simulink model "gatorKator_spectrum_visualization"  (Simulink 7.7)
settings: Solver=FixedStepDiscrete  StartTime=21e-3  StopTime=inf  RelTol=1e-3
undefined symbols (not defined in the file or in its folder): jet
libraries: dspsnks4 x5, dspspect3 x2, dspmtrx3 x2, dspmathops x2, commchan3 x1, dsparch4 x1, dspsrcs4 x1, dspstat3 x1, dspindex x1
settings Model: Creator=staticd  LastModifiedBy=staticd

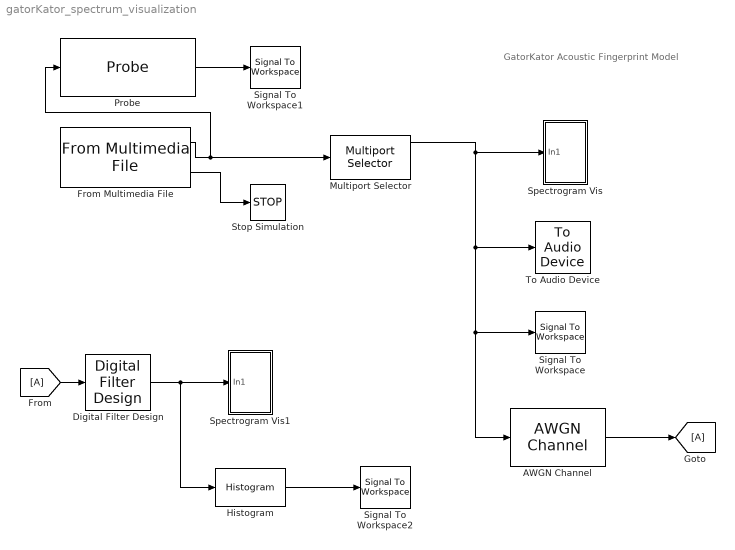
== system gatorKator_spectrum_visualization ==
  note: GatorKator Acoustic Fingerprint Model
  AWGN Channel : commchan3/AWGN Channel  SystemSampleTime=-1  InputProcessing=Columns as channels (frame based)  seed=67  noiseMode="Signal to noise ratio  (SNR)"  EbNodB=10  EsNodB=10  SNRdB=-20  bitsPerSym=1  Ps=1  Tsym=1  variance=1
  Digital Filter Design : dsparch4/Digital Filter Design  SystemSampleTime=-1  mwdsp_browser_bugfix_var=off
  From Multimedia File : dspsrcs4/From Multimedia File  inputFilename=C:\Users\staticd\Documents\My Dropbox\forLeo (2)\project\sample_data\deep_growl_converted.wav  loop=on  numPlays=inf  outputStreams=Audio only  videoDataType=single  audioDataType=double  inheritSampleTime=on  userDefinedSampleTime=1/30  noAudioOutput=off  isIntensityVideo=off  fourcc=RGB  colorVideoFormat=Separate color signals  outputEOF=on  dataOrg=Column-major  audioFrameSize=1024  computeAudioFrameSize=off
  Histogram : dspstat3/Histogram  umin=-1  umax=1  nbins=1e3  normalized=off  run=off  reset=on  trigtype=None  operateOver=Entire input  Dimension=1  colComp=on  roundingMode=Floor  overflowMode=off
  Multiport Selector : dspindex/Multiport Selector  rowsOrCols=Columns  idxCellArray={ 4, [1:2 5], [7; 8], 10:-1:6 }  idxErrMode=Clip Index
  Probe : Probe  ProbeWidth=off  ProbeComplexSignal=off
  Signal To Workspace : SignalToWorkspace  VariableName=yout  SaveFormat=Array  Save2DMode=2-D array (concatenate along first dimension)
      settings: CopyFcn=dspblkcopystw(gcbh);
  Signal To Workspace1 : SignalToWorkspace  VariableName=T  SaveFormat=Array  Save2DMode=2-D array (concatenate along first dimension)
      settings: CopyFcn=dspblkcopystw(gcbh);
  Signal To Workspace2 : SignalToWorkspace  VariableName=T1  SaveFormat=Array  Save2DMode=2-D array (concatenate along first dimension)
      settings: CopyFcn=dspblkcopystw(gcbh);
  Spectrogram Vis : Subsystem
  Spectrogram Vis1 : Subsystem
  Stop Simulation : Stop
  To Audio Device : dspsnks4/To Audio Device  deviceName=Default  inheritSampleRate=on  sampleRate=44100  deviceDatatype=Determine from input data type  autoBufferSize=on  bufferSize=4096  queueDuration=1.0
  wires:
  From Multimedia File/1 -> Probe/1, Multiport Selector/1
  Multiport Selector/1 -> Spectrogram Vis/1(In1), To Audio Device/1, Signal To Workspace/1, AWGN Channel/1
  From Multimedia File/2 -> Stop Simulation/1
  Probe/1 -> Signal To Workspace1/1
  [A] -> Digital Filter Design/1
  Digital Filter Design/1 -> Spectrogram Vis1/1(In1), Histogram/1
  Histogram/1 -> Signal To Workspace2/1
  AWGN Channel/1 -> [A]

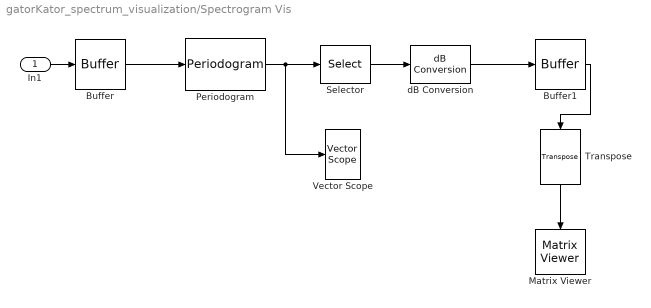
== system gatorKator_spectrum_visualization/Spectrogram Vis ==
  In1 : Inport
  Buffer : Buffer  N=256  TreatMby1Signals=One channel
  Buffer1 : Buffer  V=60  ic=-1
  Matrix Viewer : dspsnks4/Matrix Viewer  ImageParams=off  CMapStr=jet(256)  AxisColorbar=on  AxisParams=off  AxisOrigin=Lower left corner  XLabel=Time Index  YLabel=Frequency Index  ZLabel=dB Magnitude  FigPos=[50 530 1300 320]  AxisZoom=off
      settings: YMin=-80  YMax=10
  Periodogram : dspspect3/Periodogram  SystemSampleTime=-1  measurement=Power spectral density  wintype=Hamming  Rs=50  beta=5  winsamp=Periodic  inheritFFT=on  fftsize=256  navg=1  inheritTs=on  Ts=1
  Selector : Selector  InputPortWidth=256  IndexOptions=Index vector (dialog)  Indices=[1:128]  OutputSizes=1
  Transpose : dspmtrx3/Transpose  SystemSampleTime=-1  Hermitian=off  overflowFlag=off
  Vector Scope : dspsnks4/Vector Scope  ScopeProperties=on  Domain=Frequency  HorizSpan=1  DisplayProperties=off  AxisGrid=on  Memory=off  FrameNumber=on  AxisLegend=off  AxisZoom=off  OpenScopeAtSimStart=on  OpenScopeImmediately=off  FigPos=[50 110 1300 320]  AxisProperties=off  XUnits=Hertz  XRange=[0...Fs/2]  InheritXIncr=on  XIncr=1  XLabel=Time  XLimit=User-defined  XMin=0  XMax=3.5e3  XStart=0  YUnits=dB  YLabel=Magnitude, dB  LineProperties=off  XAxisParamsVer=6.9
      settings: YMin=-80  YMax=10
  dB Conversion : dspmathops/dB Conversion  SystemSampleTime=-1  dBtype=dB  intype=Power  R=1  fuzz=on
  wires:
  In1/1 -> Buffer/1
  Transpose/1 -> Matrix Viewer/1
  Buffer1/1 -> Transpose/1
  dB Conversion/1 -> Buffer1/1
  Selector/1 -> dB Conversion/1
  Periodogram/1 -> Vector Scope/1, Selector/1
  Buffer/1 -> Periodogram/1

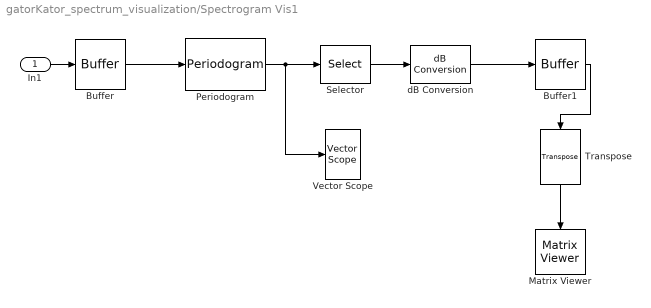
== system gatorKator_spectrum_visualization/Spectrogram Vis1 ==
  In1 : Inport
  Buffer : Buffer  N=256  TreatMby1Signals=One channel
  Buffer1 : Buffer  V=60  ic=-1
  Matrix Viewer : dspsnks4/Matrix Viewer  ImageParams=off  CMapStr=jet(256)  AxisColorbar=on  AxisParams=off  AxisOrigin=Lower left corner  XLabel=Time Index  YLabel=Frequency Index  ZLabel=dB Magnitude  FigPos=[50 530 1300 320]  AxisZoom=off
      settings: YMin=-80  YMax=10
  Periodogram : dspspect3/Periodogram  SystemSampleTime=-1  measurement=Power spectral density  wintype=Hamming  Rs=50  beta=5  winsamp=Periodic  inheritFFT=on  fftsize=256  navg=1  inheritTs=on  Ts=1
  Selector : Selector  InputPortWidth=256  IndexOptions=Index vector (dialog)  Indices=[1:128]  OutputSizes=1
  Transpose : dspmtrx3/Transpose  SystemSampleTime=-1  Hermitian=off  overflowFlag=off
  Vector Scope : dspsnks4/Vector Scope  ScopeProperties=on  Domain=Frequency  HorizSpan=1  DisplayProperties=off  AxisGrid=on  Memory=off  FrameNumber=on  AxisLegend=off  AxisZoom=off  OpenScopeAtSimStart=on  OpenScopeImmediately=off  FigPos=[50 110 1300 320]  AxisProperties=off  XUnits=Hertz  XRange=[0...Fs/2]  InheritXIncr=on  XIncr=1  XLabel=Time  XLimit=User-defined  XMin=0  XMax=3.5e3  XStart=0  YUnits=dB  YLabel=Magnitude, dB  LineProperties=off  XAxisParamsVer=6.9
      settings: YMin=-80  YMax=10
  dB Conversion : dspmathops/dB Conversion  SystemSampleTime=-1  dBtype=dB  intype=Power  R=1  fuzz=on
  wires:
  In1/1 -> Buffer/1
  Transpose/1 -> Matrix Viewer/1
  Buffer1/1 -> Transpose/1
  dB Conversion/1 -> Buffer1/1
  Selector/1 -> dB Conversion/1
  Periodogram/1 -> Vector Scope/1, Selector/1
  Buffer/1 -> Periodogram/1
